simulink subsystem "BatteryManagementSystem"  (R2023b)
settings: Solver=VariableStepAuto  StartTime=0.0  StopTime=10.0  RelTol=1e-3
undefined symbols (not defined in the file or in its folder): battery, vehicleThermal
libraries: BatteryThermalManagement x1
settings Model: DefaultTestHarness=BatteryManagementSystem_Harness  Creator=jjha  LastModifiedBy=jjha
settings OptimizationCC: ReuseModelBlockBuffer=off

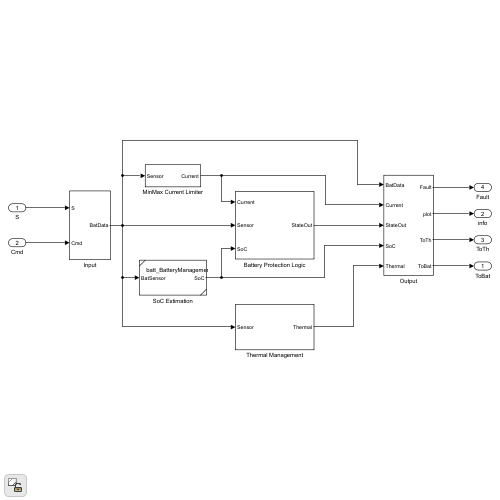
[thumbnail: Simulink's stored preview of the top-level diagram]
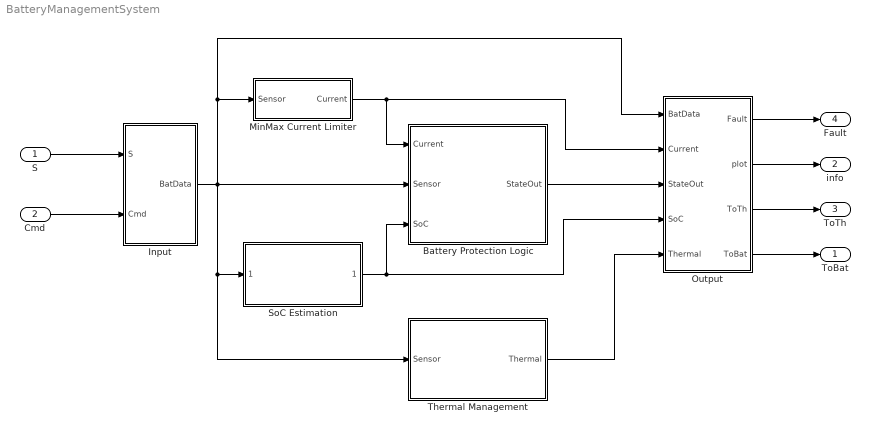
== system BatteryManagementSystem ==
  S : Inport
  Cmd : Inport  Port=2
  Battery Protection Logic : Subsystem
  Input : Subsystem
  MinMax Current Limiter : Subsystem
  Output : Subsystem
  SoC Estimation : Subsystem  ReferencedSubsystem=batt_BatteryManagementSystem_SoC
  Thermal Management : Subsystem
  ToBat : Outport
  info : Outport  Port=2
  ToTh : Outport  Port=3
  Fault : Outport  Port=4
  wires:
  Input/1(BatData) -> Battery Protection Logic/2(Sensor), SoC Estimation/1, Thermal Management/1(Sensor), Output/1(BatData), MinMax Current Limiter/1(Sensor)
  SoC Estimation/1 -> Battery Protection Logic/3(SoC), Output/4(SoC)
  Thermal Management/1(Thermal) -> Output/5(Thermal)
  MinMax Current Limiter/1(Current) -> Output/2(Current), Battery Protection Logic/1(Current)
  Battery Protection Logic/1(StateOut) -> Output/3(StateOut)
  S/1 -> Input/1(S)
  Output/1(Fault) -> Fault/1
  Output/2(plot) -> info/1
  Output/3(ToTh) -> ToTh/1
  Output/4(ToBat) -> ToBat/1
  Cmd/1 -> Input/2(Cmd)

== system BatteryManagementSystem/Battery Protection Logic ==
  Current : Inport
  Sensor : Inport  Port=2
  SoC : Inport  Port=3
  State Flow Logic : Subsystem  mask{MinVoltLmt=battery.MinVoltLmt, MaxVoltLmt=battery.MaxVoltLmt, VoltOffset=battery.VoltOffset, CurrOffset=battery.CurrOffset, MinThLmt=battery.MinThLmt, MaxThLmt=battery.MaxThLmt}
      mask prompts: MinVoltLmt "Minimum Voltage Limit"; MaxVoltLmt "Maximum Voltage Limit"; VoltOffset "Voltage fault offset"; CurrOffset "Current fault offset"; MinThLmt "Min cell temp"; MaxThLmt "Max cell temp"
      mask DialogControl ParameterGroupVar Prompt: Battery Fault Parameters
  Stateflow Input : Subsystem
  StateOut : Outport
  wires:
  State Flow Logic/1(StateOut) -> StateOut/1
  Stateflow Input/1(StateInput) -> State Flow Logic/1(StateInput)
  SoC/1 -> Stateflow Input/1(SoC)
  Current/1 -> Stateflow Input/2(Current)
  Sensor/1 -> Stateflow Input/3(Sensor)

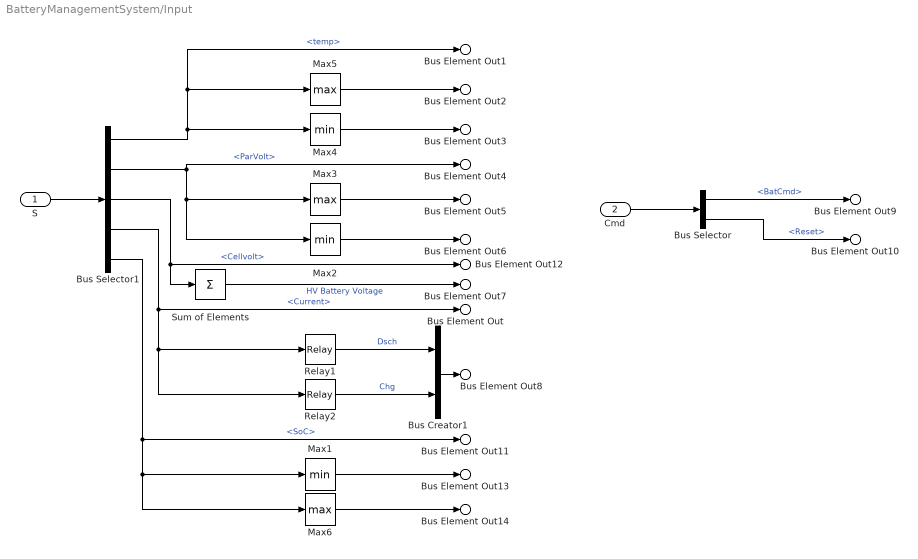
== system BatteryManagementSystem/Input ==
  S : Inport
  Cmd : Inport  Port=2
  Bus Creator1 : BusCreator  Inputs=2
  Bus Selector : BusSelector  OutputSignals=BatCmd,Reset
  Bus Selector1 : BusSelector  OutputSignals=temp,ParVolt,Cellvolt,Current,SoC
  Max1 : MinMax  ZeroCross=off
  Max2 : MinMax  ZeroCross=off
  Max3 : MinMax  Function=max  ZeroCross=off
  Max4 : MinMax  ZeroCross=off
  Max5 : MinMax  Function=max  ZeroCross=off
  Max6 : MinMax  Function=max  ZeroCross=off
  Relay1 : Relay  OnSwitchValue=0  OffSwitchValue=-5  OnOutputValue=0  OffOutputValue=1  ZeroCross=off
  Relay2 : Relay  OnSwitchValue=5  OffSwitchValue=0  ZeroCross=off
  Sum of Elements : Sum  Inputs=+
  Bus Element Out : Outport  PortName=BatData  Element=Cur
  Bus Element Out1 : Outport  PortName=BatData  Element=CellTemp
  Bus Element Out2 : Outport  PortName=BatData  Element=CellTempMax
  Bus Element Out3 : Outport  PortName=BatData  Element=CellTempMin
  Bus Element Out4 : Outport  PortName=BatData  Element=CellVolt
  Bus Element Out5 : Outport  PortName=BatData  Element=CellVoltMax
  Bus Element Out6 : Outport  PortName=BatData  Element=CellVoltMin
  Bus Element Out7 : Outport  PortName=BatData  Element=BatVolt
  Bus Element Out8 : Outport  PortName=BatData  Element=CurDir
  Bus Element Out11 : Outport  PortName=BatData  Element=SoC
  Bus Element Out12 : Outport  PortName=BatData  Element=BatParVolt
  Bus Element Out13 : Outport  PortName=BatData  Element=minSoC
  Bus Element Out14 : Outport  PortName=BatData  Element=maxSoC
  Bus Element Out9 : Outport  PortName=BatData  Element=BatCmd
  Bus Element Out10 : Outport  PortName=BatData  Element=Reset
  wires:
  Bus Selector/2 -> Bus Element Out10/1  "<Reset>"
  Cmd/1 -> Bus Selector/1
  Bus Selector/1 -> Bus Element Out9/1  "<BatCmd>"
  Bus Selector1/5 -> Bus Element Out11/1, Max1/1, Max6/1  "<SoC>"
  Bus Selector1/3 -> Sum of Elements/1, Bus Element Out12/1  "<Cellvolt>"
  Relay1/1 -> Bus Creator1/1  "Dsch"
  Bus Selector1/1 -> Bus Element Out1/1, Max5/1, Max4/1  "<temp>"
  Bus Selector1/4 -> Bus Element Out/1, Relay1/1, Relay2/1  "<Current>"
  Sum of Elements/1 -> Bus Element Out7/1  "HV Battery Voltage"
  S/1 -> Bus Selector1/1
  Bus Selector1/2 -> Bus Element Out4/1, Max3/1, Max2/1  "<ParVolt>"
  Max5/1 -> Bus Element Out2/1
  Max4/1 -> Bus Element Out3/1
  Max3/1 -> Bus Element Out5/1
  Max2/1 -> Bus Element Out6/1
  Bus Creator1/1 -> Bus Element Out8/1
  Relay2/1 -> Bus Creator1/2  "Chg"
  Max1/1 -> Bus Element Out13/1
  Max6/1 -> Bus Element Out14/1

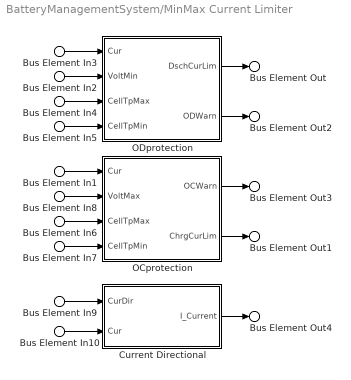
== system BatteryManagementSystem/MinMax Current Limiter ==
  Bus Element In3 : Inport  PortName=Sensor  Element=Cur
  Bus Element In1 : Inport  PortName=Sensor  Element=Cur
  Bus Element In10 : Inport  PortName=Sensor  Element=Cur
  Bus Element In2 : Inport  PortName=Sensor  Element=CellVoltMin
  Bus Element In8 : Inport  PortName=Sensor  Element=CellVoltMax
  Bus Element In9 : Inport  PortName=Sensor  Element=CurDir
  Bus Element In5 : Inport  PortName=Sensor  Element=CellTempMin
  Bus Element In7 : Inport  PortName=Sensor  Element=CellTempMin
  Bus Element In4 : Inport  PortName=Sensor  Element=CellTempMax
  Bus Element In6 : Inport  PortName=Sensor  Element=CellTempMax
  Current Directional : Subsystem
  OCprotection : Subsystem
  ODprotection : Subsystem
  Bus Element Out : Outport  PortName=Current  Element=CurDchLmt
  Bus Element Out1 : Outport  PortName=Current  Element=CurChgLmt
  Bus Element Out2 : Outport  PortName=Current  Element=CurDchWarn
  Bus Element Out3 : Outport  PortName=Current  Element=CurChgWarn
  Bus Element Out4 : Outport  PortName=Current  Element=CurChgDchg
  wires:
  ODprotection/2(ODWarn) -> Bus Element Out2/1
  Bus Element In8/1 -> OCprotection/2(VoltMax)
  Bus Element In2/1 -> ODprotection/2(VoltMin)
  OCprotection/1(OCWarn) -> Bus Element Out3/1
  Bus Element In6/1 -> OCprotection/3(CellTpMax)
  Bus Element In7/1 -> OCprotection/4(CellTpMin)
  Bus Element In9/1 -> Current Directional/1(CurDir)
  Bus Element In4/1 -> ODprotection/3(CellTpMax)
  Bus Element In5/1 -> ODprotection/4(CellTpMin)
  ODprotection/1(DschCurLim) -> Bus Element Out/1
  OCprotection/2(ChrgCurLim) -> Bus Element Out1/1
  Bus Element In3/1 -> ODprotection/1(Cur)
  Bus Element In1/1 -> OCprotection/1(Cur)
  Current Directional/1(I_Current) -> Bus Element Out4/1
  Bus Element In10/1 -> Current Directional/2(Cur)

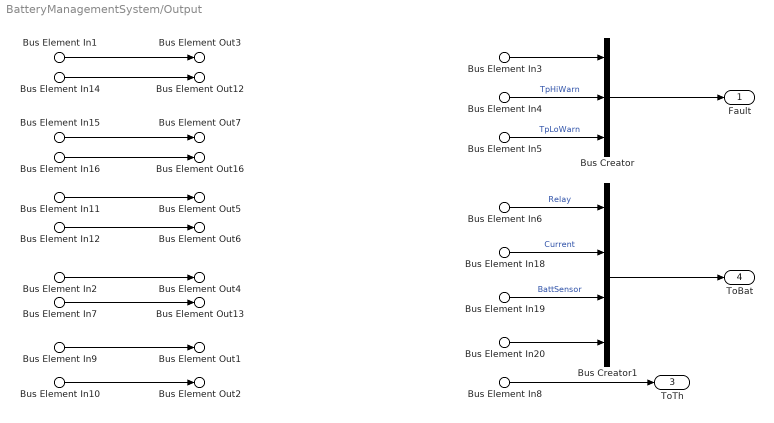
== system BatteryManagementSystem/Output ==
  Bus Element In19 : Inport  PortName=BatData
  Bus Element In9 : Inport  PortName=BatData  Element=Cur
  Bus Element In10 : Inport  PortName=BatData  Element=BatVolt
  Bus Element In11 : Inport  PortName=BatData  Element=CellTempMax
  Bus Element In12 : Inport  PortName=BatData  Element=CellTempMin
  Bus Element In18 : Inport  Port=2  PortName=Current
  Bus Element In2 : Inport  Port=2  PortName=Current  Element=CurChgLmt
  Bus Element In7 : Inport  Port=2  PortName=Current  Element=CurDchLmt
  Bus Element In3 : Inport  Port=3  PortName=StateOut  Element=Fault
  Bus Element In6 : Inport  Port=3  PortName=StateOut  Element=RelayRq
  Bus Element In20 : Inport  Port=3  PortName=StateOut  Element=BatSt
  Bus Element In1 : Inport  Port=4  PortName=SoC  Element=CellSoCmax
  Bus Element In14 : Inport  Port=4  PortName=SoC  Element=CellSoCmin
  Bus Element In8 : Inport  Port=5  PortName=Thermal
  Bus Element In{4..5,15..16} (4 alike) : Inport  Port=5  PortName=Thermal  Element=TpHiWarning
  Bus Creator : BusCreator  Inputs=3
  Bus Creator1 : BusCreator  Inputs=4
  Fault : Outport
  Bus Element Out3 : Outport  Port=2  PortName=plot  Element=SoCMax
  Bus Element Out4 : Outport  Port=2  PortName=plot  Element=CurChgLmt
  Bus Element Out7 : Outport  Port=2  PortName=plot  Element=HiThWarn
  Bus Element Out12 : Outport  Port=2  PortName=plot  Element=SoCMin
  Bus Element Out13 : Outport  Port=2  PortName=plot  Element=CurDchgLmt
  Bus Element Out16 : Outport  Port=2  PortName=plot  Element=LoThWarn
  Bus Element Out1 : Outport  Port=2  PortName=plot  Element=Cur
  Bus Element Out2 : Outport  Port=2  PortName=plot  Element=BatVolt
  Bus Element Out5 : Outport  Port=2  PortName=plot  Element=TpMax
  Bus Element Out6 : Outport  Port=2  PortName=plot  Element=TpMin
  ToTh : Outport  Port=3
  ToBat : Outport  Port=4
  wires:
  Bus Element In8/1 -> ToTh/1
  Bus Creator/1 -> Fault/1
  Bus Creator1/1 -> ToBat/1
  Bus Element In18/1 -> Bus Creator1/2  "Current"
  Bus Element In12/1 -> Bus Element Out6/1
  Bus Element In11/1 -> Bus Element Out5/1
  Bus Element In10/1 -> Bus Element Out2/1
  Bus Element In9/1 -> Bus Element Out1/1
  Bus Element In6/1 -> Bus Creator1/1  "Relay"
  Bus Element In5/1 -> Bus Creator/3  "TpLoWarn"
  Bus Element In4/1 -> Bus Creator/2  "TpHiWarn"
  Bus Element In3/1 -> Bus Creator/1
  Bus Element In14/1 -> Bus Element Out12/1
  Bus Element In2/1 -> Bus Element Out4/1
  Bus Element In1/1 -> Bus Element Out3/1
  Bus Element In7/1 -> Bus Element Out13/1
  Bus Element In15/1 -> Bus Element Out7/1
  Bus Element In16/1 -> Bus Element Out16/1
  Bus Element In19/1 -> Bus Creator1/3  "BattSensor"
  Bus Element In20/1 -> Bus Creator1/4

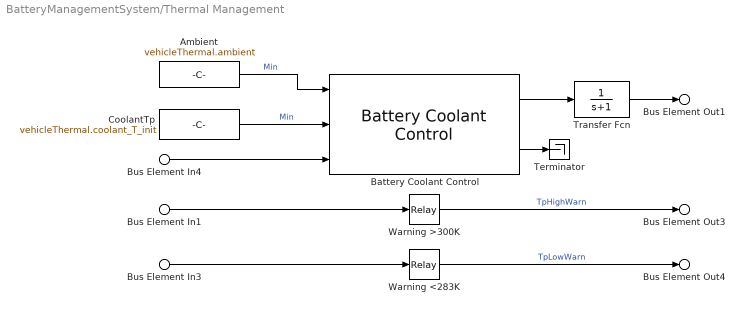
== system BatteryManagementSystem/Thermal Management ==
  Bus Element In3 : Inport  PortName=Sensor  Element=CellTempMin
  Bus Element In1 : Inport  PortName=Sensor  Element=CellTempMax
  Bus Element In4 : Inport  PortName=Sensor  Element=CellTemp
  Ambient : Constant  Value=vehicleThermal.ambient
  Battery Coolant Control : BatteryThermalManagement/Battery Coolant Control  ControlStrategy=ON-OFF control  TempOn=battery.CoolantSwitchOnTp  TempOff=battery.CoolantSwitchOffTp  c=0.1  FlowRateStep=0.2
      settings: LibrarySourceBlock=batt_sl_lib/Thermal Management/Battery Coolant Control
  CoolantTp : Constant  Value=vehicleThermal.coolant_T_init
  Terminator : Terminator
  Transfer Fcn : TransferFcn  Denominator=[1 1]
  Warning <283K : Relay  OnSwitchValue=290  OffSwitchValue=283  OnOutputValue=0  OffOutputValue=1  ZeroCross=off
  Warning >300K : Relay  OnSwitchValue=320  OffSwitchValue=310  ZeroCross=off
  Bus Element Out1 : Outport  PortName=Thermal  Element=CoolFlow
  Bus Element Out3 : Outport  PortName=Thermal  Element=TpHiWarning
  Bus Element Out4 : Outport  PortName=Thermal  Element=TpLoWarning
  wires:
  Battery Coolant Control/2 -> Terminator/1
  Bus Element In4/1 -> Battery Coolant Control/3
  Transfer Fcn/1 -> Bus Element Out1/1
  CoolantTp/1 -> Battery Coolant Control/2  "Min"
  Ambient/1 -> Battery Coolant Control/1  "Min"
  Bus Element In3/1 -> Warning <283K/1
  Bus Element In1/1 -> Warning >300K/1
  Warning <283K/1 -> Bus Element Out4/1  "TpLowWarn"
  Warning >300K/1 -> Bus Element Out3/1  "TpHighWarn"
  Battery Coolant Control/1 -> Transfer Fcn/1

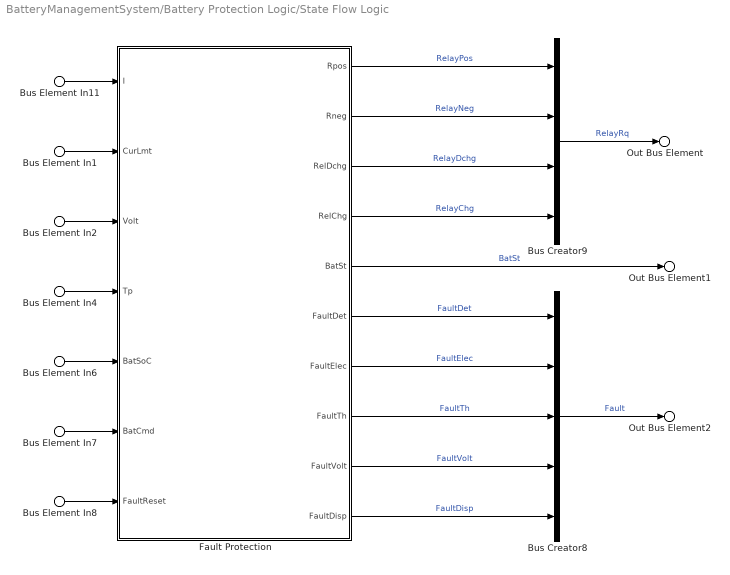
== system BatteryManagementSystem/Battery Protection Logic/State Flow Logic ==
  Bus Element In11 : Inport  PortName=StateInput  Element=Current
  Bus Element In1 : Inport  PortName=StateInput  Element=CurLmt
  Bus Element In2 : Inport  PortName=StateInput  Element=Volt
  Bus Element In4 : Inport  PortName=StateInput  Element=Tp
  Bus Element In6 : Inport  PortName=StateInput  Element=BatSoC
  Bus Element In7 : Inport  PortName=StateInput  Element=BatCmd
  Bus Element In8 : Inport  PortName=StateInput  Element=FaultReset
  Bus Creator8 : BusCreator  Inputs=5
  Bus Creator9 : BusCreator  Inputs=4
  Fault Protection : Stateflow chart  TreatAsAtomicUnit=on
      settings: PortSchema="{\"entries\":[{\"content\":{\"sides\":[{\"content\":{\"connectorIds\":[\"In1\",\"In2\",\"In3\",\"In4\",\"In5\",\"In6\",\"In7\"]},\"type\":\"ConnectorPlacement.EquallySpacedRectSide\",\"uuid\":\"7222f55a-2aef-4ca8-adbd-e86ed030f82f\"},{\"content\":{\"connectorIds\":[\"Out5\",\"Out6\",\"Out10\",\"Out9\",\"Out4\",\"Out1\",\"Out2\",\"Out3\",\"Out7\",\"Out8\"],\"side\":\"RIGHT\"},\"type\":\"ConnectorPlacement.EquallySpacedRectSide\",\"uuid\":\"bfa2f4e3-3563-4466-8725-57bf2336ec66\"},{\"content\":{\"connectorIds\":[],\"side\":\"TOP\"},\"type\":\"ConnectorPlacement.EquallySpacedRectSide\",\"uuid\":\"7b1e9a44-7135-4c45-bb2b-0152be29b46d\"}]},\"type\":\"ConnectorPlacement.EquallySpacedConnector\",\"uuid\":\"80032a24-3823-40c6-b797-ffbc29f7d345\"}],\"packageUris\":[\"http://schema.mathworks.com/mf0/Connector/R2020b\"],\"version\":\"1.0\"}"
  Out Bus Element : Outport  PortName=StateOut  Element=RelayRq
  Out Bus Element1 : Outport  PortName=StateOut  Element=BatSt
  Out Bus Element2 : Outport  PortName=StateOut  Element=Fault
  wires:
  Fault Protection/4(BatSt) -> Out Bus Element1/1  "BatSt"
  Fault Protection/9(RelChg) -> Bus Creator9/4  "RelayChg"
  Fault Protection/10(RelDchg) -> Bus Creator9/3  "RelayDchg"
  Fault Protection/6(Rneg) -> Bus Creator9/2  "RelayNeg"
  Fault Protection/5(Rpos) -> Bus Creator9/1  "RelayPos"
  Bus Element In7/1 -> Fault Protection/6(BatCmd)
  Bus Element In8/1 -> Fault Protection/7(FaultReset)
  Bus Element In2/1 -> Fault Protection/3(Volt)
  Bus Element In1/1 -> Fault Protection/2(CurLmt)
  Bus Element In11/1 -> Fault Protection/1(I)
  Bus Element In4/1 -> Fault Protection/4(Tp)
  Bus Element In6/1 -> Fault Protection/5(BatSoC)
  Bus Creator9/1 -> Out Bus Element/1  "RelayRq"
  Bus Creator8/1 -> Out Bus Element2/1  "Fault"
  Fault Protection/2(FaultElec) -> Bus Creator8/2  "FaultElec"
  Fault Protection/3(FaultTh) -> Bus Creator8/3  "FaultTh"
  Fault Protection/7(FaultVolt) -> Bus Creator8/4  "FaultVolt"
  Fault Protection/8(FaultDisp) -> Bus Creator8/5  "FaultDisp"
  Fault Protection/1(FaultDet) -> Bus Creator8/1  "FaultDet"

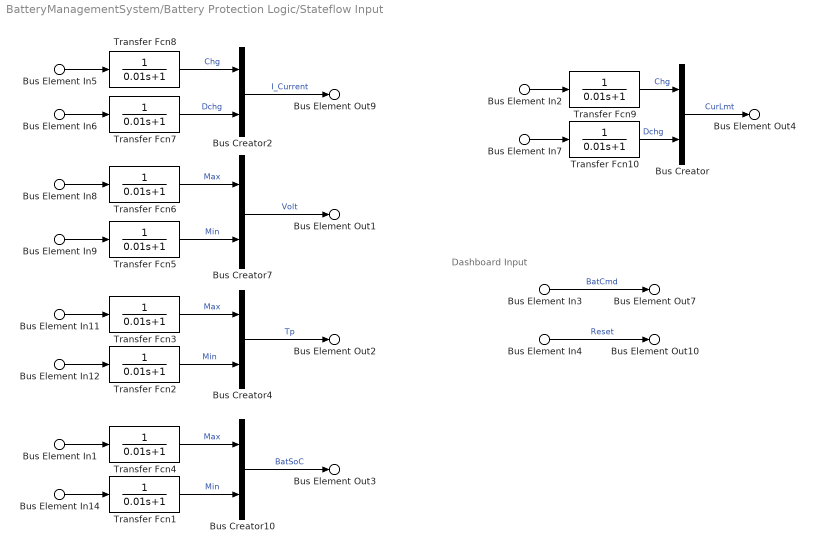
== system BatteryManagementSystem/Battery Protection Logic/Stateflow Input ==
  note: Dashboard Input
  Bus Element In1 : Inport  PortName=SoC  Element=CellSoCmax
  Bus Element In14 : Inport  PortName=SoC  Element=CellSoCmin
  Bus Element In2 : Inport  Port=2  PortName=Current  Element=CurChgLmt
  Bus Element In7 : Inport  Port=2  PortName=Current  Element=CurDchLmt
  Bus Element In5 : Inport  Port=2  PortName=Current  Element=CurChgDchg.Chg
  Bus Element In6 : Inport  Port=2  PortName=Current  Element=CurChgDchg.Dchg
  Bus Element In8 : Inport  Port=3  PortName=Sensor  Element=CellVoltMax
  Bus Element In9 : Inport  Port=3  PortName=Sensor  Element=CellVoltMin
  Bus Element In11 : Inport  Port=3  PortName=Sensor  Element=CellTempMax
  Bus Element In12 : Inport  Port=3  PortName=Sensor  Element=CellTempMin
  Bus Element In3 : Inport  Port=3  PortName=Sensor  Element=BatCmd
  Bus Element In4 : Inport  Port=3  PortName=Sensor  Element=Reset
  Bus Creator : BusCreator  Inputs=2  OutDataTypeStr=Bus: I_Current
  Bus Creator10 : BusCreator  Inputs=2  OutDataTypeStr=Bus: MaxMinLimit
  Bus Creator2 : BusCreator  Inputs=2  OutDataTypeStr=Bus: I_Current
  Bus Creator4 : BusCreator  Inputs=2  OutDataTypeStr=Bus: MaxMinLimit
  Bus Creator7 : BusCreator  Inputs=2  OutDataTypeStr=Bus: CellVoltage  NonVirtualBus=on
  Transfer Fcn{1..10} (10 alike) : TransferFcn  Denominator=[0.01 1]
  Bus Element Out9 : Outport  PortName=StateInput  Element=Current
  Bus Element Out1 : Outport  PortName=StateInput  Element=Volt
  Bus Element Out2 : Outport  PortName=StateInput  Element=Tp
  Bus Element Out3 : Outport  PortName=StateInput  Element=BatSoC
  Bus Element Out4 : Outport  PortName=StateInput  Element=CurLmt
  Bus Element Out7 : Outport  PortName=StateInput  Element=BatCmd
  Bus Element Out10 : Outport  PortName=StateInput  Element=FaultReset
  wires:
  Transfer Fcn10/1 -> Bus Creator/2  "Dchg"
  Transfer Fcn9/1 -> Bus Creator/1  "Chg"
  Transfer Fcn7/1 -> Bus Creator2/2  "Dchg"
  Transfer Fcn8/1 -> Bus Creator2/1  "Chg"
  Transfer Fcn6/1 -> Bus Creator7/1  "Max"
  Transfer Fcn5/1 -> Bus Creator7/2  "Min"
  Transfer Fcn3/1 -> Bus Creator4/1  "Max"
  Transfer Fcn2/1 -> Bus Creator4/2  "Min"
  Transfer Fcn1/1 -> Bus Creator10/2  "Min"
  Transfer Fcn4/1 -> Bus Creator10/1  "Max"
  Bus Element In7/1 -> Transfer Fcn10/1
  Bus Element In2/1 -> Transfer Fcn9/1
  Bus Creator7/1 -> Bus Element Out1/1  "Volt"
  Bus Creator2/1 -> Bus Element Out9/1  "I_Current"
  Bus Creator4/1 -> Bus Element Out2/1  "Tp"
  Bus Element In3/1 -> Bus Element Out7/1  "BatCmd"
  Bus Element In4/1 -> Bus Element Out10/1  "Reset"
  Bus Element In14/1 -> Transfer Fcn1/1
  Bus Element In1/1 -> Transfer Fcn4/1
  Bus Element In6/1 -> Transfer Fcn7/1
  Bus Element In5/1 -> Transfer Fcn8/1
  Bus Creator10/1 -> Bus Element Out3/1  "BatSoC"
  Bus Element In11/1 -> Transfer Fcn3/1
  Bus Creator/1 -> Bus Element Out4/1  "CurLmt"
  Bus Element In9/1 -> Transfer Fcn5/1
  Bus Element In8/1 -> Transfer Fcn6/1
  Bus Element In12/1 -> Transfer Fcn2/1

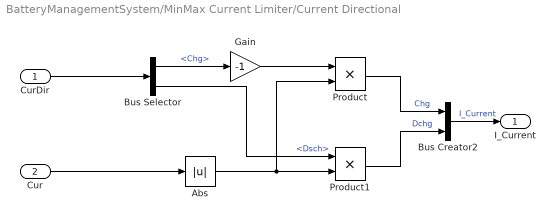
== system BatteryManagementSystem/MinMax Current Limiter/Current Directional ==
  CurDir : Inport
  Cur : Inport  Port=2
  Abs : Abs  ZeroCross=off  SaturateOnIntegerOverflow=off
  Bus Creator2 : BusCreator  Inputs=2  OutDataTypeStr=Bus: I_Current
  Bus Selector : BusSelector  OutputSignals=Chg,Dsch
  Gain : Gain  Gain=-1
  Product : Product
  Product1 : Product
  I_Current : Outport
  wires:
  Gain/1 -> Product/1
  Cur/1 -> Abs/1
  Abs/1 -> Product/2, Product1/2
  CurDir/1 -> Bus Selector/1
  Bus Selector/1 -> Gain/1  "<Chg>"
  Bus Selector/2 -> Product1/1  "<Dsch>"
  Product/1 -> Bus Creator2/1  "Chg"
  Bus Creator2/1 -> I_Current/1  "I_Current"
  Product1/1 -> Bus Creator2/2  "Dchg"

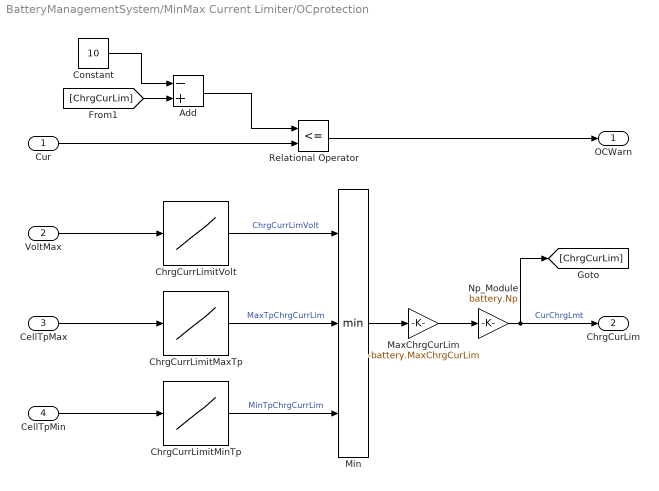
== system BatteryManagementSystem/MinMax Current Limiter/OCprotection ==
  Cur : Inport
  VoltMax : Inport  Port=2
  CellTpMax : Inport  Port=3
  CellTpMin : Inport  Port=4
  Add : Sum  Inputs=-+
  ChrgCurrLimitMaxTp : Lookup_n-D  NumberOfTableDimensions=1  BreakpointsForDimension1="single([313  318  323  328 333])"  BreakpointsForDimension3=[5, 7]  Table=single([1.0 0.8 0.5 0.3 0])  ExtrapMethod=Clip  UseLastTableValue=on  InternalRulePriority=Speed  RndMeth=Simplest
  ChrgCurrLimitMinTp : Lookup_n-D  NumberOfTableDimensions=1  BreakpointsForDimension1=single([258 263 268 273 278 283 288])  BreakpointsForDimension3=[5, 7]  Table="single([0.1 0.2  0.3 0.3 0.5 1.0 1.0])"  ExtrapMethod=Clip  UseLastTableValue=on  InternalRulePriority=Speed  RndMeth=Simplest
  ChrgCurrLimitVolt : Lookup_n-D  NumberOfTableDimensions=1  BreakpointsForDimension1=single([3.9 4.0 4.15 4.2])  BreakpointsForDimension3=[5, 7]  Table="single([1.0 0.8 0.3  0.3])"  ExtrapMethod=Clip  UseLastTableValue=on  InternalRulePriority=Speed  RndMeth=Simplest
  Constant : Constant  Value=10
  MaxChrgCurLim : Gain  Gain=-battery.MaxChrgCurLim
  Min : MinMax  Inputs=3
  Np_Module : Gain  Gain=battery.Np
  Relational Operator : RelationalOperator  Operator=<=  OutDataTypeStr=boolean  RndMeth=Simplest  InputSameDT=off
  OCWarn : Outport
  ChrgCurLim : Outport  Port=2
  wires:
  Add/1 -> Relational Operator/1
  Constant/1 -> Add/1
  VoltMax/1 -> ChrgCurrLimitVolt/1
  ChrgCurrLimitVolt/1 -> Min/1  "ChrgCurrLimVolt"
  MaxChrgCurLim/1 -> Np_Module/1
  Np_Module/1 -> ChrgCurLim/1, [ChrgCurLim]  "CurChrgLmt"
  CellTpMax/1 -> ChrgCurrLimitMaxTp/1
  CellTpMin/1 -> ChrgCurrLimitMinTp/1
  ChrgCurrLimitMaxTp/1 -> Min/2  "MaxTpChrgCurrLim"
  ChrgCurrLimitMinTp/1 -> Min/3  "MinTpChrgCurrLim"
  Min/1 -> MaxChrgCurLim/1
  Cur/1 -> Relational Operator/2
  [ChrgCurLim] -> Add/2
  Relational Operator/1 -> OCWarn/1

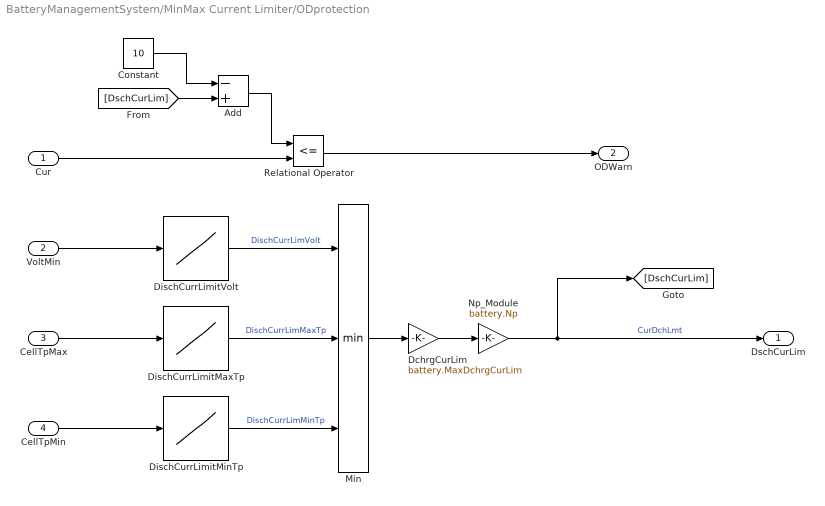
== system BatteryManagementSystem/MinMax Current Limiter/ODprotection ==
  Cur : Inport
  VoltMin : Inport  Port=2
  CellTpMax : Inport  Port=3
  CellTpMin : Inport  Port=4
  Add : Sum  Inputs=-+
  Constant : Constant  Value=10
  DchrgCurLim : Gain  Gain=battery.MaxDchrgCurLim
  DischCurrLimitMaxTp : Lookup_n-D  NumberOfTableDimensions=1  BreakpointsForDimension1=single([313, 318, 323, 333])  BreakpointsForDimension3=[5, 7]  Table=single([1, 0.5, 0.3, 0])  ExtrapMethod=Clip  UseLastTableValue=on  InternalRulePriority=Speed  RndMeth=Simplest
  DischCurrLimitMinTp : Lookup_n-D  NumberOfTableDimensions=1  BreakpointsForDimension1="single([263, 268,    273,   278, 283, 288, 293])"  BreakpointsForDimension3=[5, 7]  Table="single([0,  0.2, 0.3, 0.5, 0.75, 1, 1])"  ExtrapMethod=Clip  UseLastTableValue=on  InternalRulePriority=Speed  RndMeth=Simplest
  DischCurrLimitVolt : Lookup_n-D  NumberOfTableDimensions=1  BreakpointsForDimension1=single([2.5;3;3.5;4.2])  BreakpointsForDimension3=[5, 7]  Table=single([0 0.25 0.5 0.75])  ExtrapMethod=Clip  UseLastTableValue=on  InternalRulePriority=Speed  RndMeth=Simplest
  Min : MinMax  Inputs=3
  Np_Module : Gain  Gain=battery.Np
  Relational Operator : RelationalOperator  Operator=<=  OutDataTypeStr=boolean  RndMeth=Simplest  InputSameDT=off
  DschCurLim : Outport
  ODWarn : Outport  Port=2
  wires:
  Constant/1 -> Add/1
  Add/1 -> Relational Operator/1
  Relational Operator/1 -> ODWarn/1
  [DschCurLim] -> Add/2
  Cur/1 -> Relational Operator/2
  Min/1 -> DchrgCurLim/1
  DischCurrLimitMinTp/1 -> Min/3  "DischCurrLimMinTp"
  DischCurrLimitMaxTp/1 -> Min/2  "DischCurrLimMaxTp"
  CellTpMax/1 -> DischCurrLimitMaxTp/1
  Np_Module/1 -> [DschCurLim], DschCurLim/1  "CurDchLmt"
  DchrgCurLim/1 -> Np_Module/1
  DischCurrLimitVolt/1 -> Min/1  "DischCurrLimVolt"
  VoltMin/1 -> DischCurrLimitVolt/1
  CellTpMin/1 -> DischCurrLimitMinTp/1

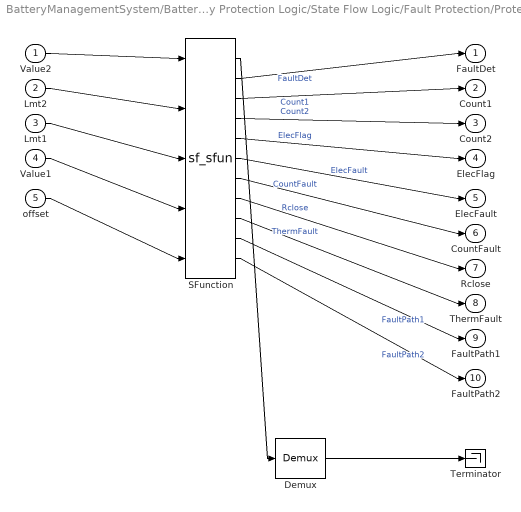
== system BatteryManagementSystem/Battery Protection Logic/State Flow Logic/Fault Protection/Protection.CurrFault ==
  Value2 : Inport
  Lmt2 : Inport  Port=2
  Lmt1 : Inport  Port=3
  Value1 : Inport  Port=4
  offset : Inport  Port=5
  " Demux " : Demux  Outputs=1
  " SFunction " : S-Function  Tag=Stateflow S-Function 3  FunctionName=sf_sfun  PortCounts=[5 11]  SFunctionDeploymentMode=off  EnableBusSupport=off
  " Terminator " : Terminator
  FaultDet : Outport
  Count1 : Outport  Port=2
  Count2 : Outport  Port=3
  ElecFlag : Outport  Port=4
  ElecFault : Outport  Port=5
  CountFault : Outport  Port=6
  Rclose : Outport  Port=7
  ThermFault : Outport  Port=8
  FaultPath1 : Outport  Port=9
  FaultPath2 : Outport  Port=10
  wires:
  Value2/1 -> " SFunction "/1
  Lmt2/1 -> " SFunction "/2
  Lmt1/1 -> " SFunction "/3
  Value1/1 -> " SFunction "/4
  offset/1 -> " SFunction "/5
  " SFunction "/2 -> FaultDet/1  "FaultDet"
  " SFunction "/3 -> Count1/1  "Count1"
  " SFunction "/4 -> Count2/1  "Count2"
  " SFunction "/5 -> ElecFlag/1  "ElecFlag"
  " SFunction "/6 -> ElecFault/1  "ElecFault"
  " SFunction "/7 -> CountFault/1  "CountFault"
  " SFunction "/8 -> Rclose/1  "Rclose"
  " SFunction "/9 -> ThermFault/1  "ThermFault"
  " SFunction "/10 -> FaultPath1/1  "FaultPath1"
  " SFunction "/11 -> FaultPath2/1  "FaultPath2"
  " Demux "/1 -> " Terminator "/1
  " SFunction "/1 -> " Demux "/1

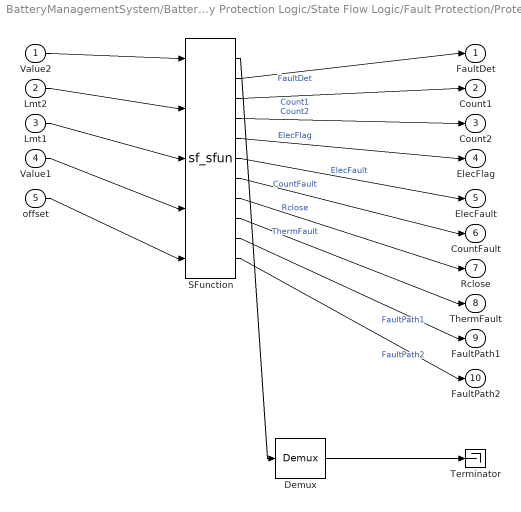
== system BatteryManagementSystem/Battery Protection Logic/State Flow Logic/Fault Protection/Protection.VoltageFault ==
  Value2 : Inport
  Lmt2 : Inport  Port=2
  Lmt1 : Inport  Port=3
  Value1 : Inport  Port=4
  offset : Inport  Port=5
  " Demux " : Demux  Outputs=1
  " SFunction " : S-Function  Tag=Stateflow S-Function 5  FunctionName=sf_sfun  PortCounts=[5 11]  SFunctionDeploymentMode=off  EnableBusSupport=off
  " Terminator " : Terminator
  FaultDet : Outport
  Count1 : Outport  Port=2
  Count2 : Outport  Port=3
  ElecFlag : Outport  Port=4
  ElecFault : Outport  Port=5
  CountFault : Outport  Port=6
  Rclose : Outport  Port=7
  ThermFault : Outport  Port=8
  FaultPath1 : Outport  Port=9
  FaultPath2 : Outport  Port=10
  wires:
  Value2/1 -> " SFunction "/1
  Lmt2/1 -> " SFunction "/2
  Lmt1/1 -> " SFunction "/3
  Value1/1 -> " SFunction "/4
  offset/1 -> " SFunction "/5
  " SFunction "/2 -> FaultDet/1  "FaultDet"
  " SFunction "/3 -> Count1/1  "Count1"
  " SFunction "/4 -> Count2/1  "Count2"
  " SFunction "/5 -> ElecFlag/1  "ElecFlag"
  " SFunction "/6 -> ElecFault/1  "ElecFault"
  " SFunction "/7 -> CountFault/1  "CountFault"
  " SFunction "/8 -> Rclose/1  "Rclose"
  " SFunction "/9 -> ThermFault/1  "ThermFault"
  " SFunction "/10 -> FaultPath1/1  "FaultPath1"
  " SFunction "/11 -> FaultPath2/1  "FaultPath2"
  " Demux "/1 -> " Terminator "/1
  " SFunction "/1 -> " Demux "/1

== system BatteryManagementSystem/Battery Protection Logic/State Flow Logic/Fault Protection/Relay_Charge ==
  " Demux " : Demux  Outputs=1
  " Ground " : Ground
  " SFunction " : S-Function  Tag=Stateflow S-Function 6  FunctionName=sf_sfun  PortCounts=[1 5]  SFunctionDeploymentMode=off  EnableBusSupport=off
  " Terminator " : Terminator
  RelClosing : Outport
  RelClose : Outport  Port=2
  Relay : Outport  Port=3
  RelOpening : Outport  Port=4
  wires:
  " SFunction "/2 -> RelClosing/1  "RelClosing"
  " SFunction "/3 -> RelClose/1  "RelClose"
  " SFunction "/4 -> Relay/1  "Relay"
  " SFunction "/5 -> RelOpening/1  "RelOpening"
  " Ground "/1 -> " SFunction "/1
  " Demux "/1 -> " Terminator "/1
  " SFunction "/1 -> " Demux "/1

== system BatteryManagementSystem/Battery Protection Logic/State Flow Logic/Fault Protection/Relay_Discharge ==
  " Demux " : Demux  Outputs=1
  " Ground " : Ground
  " SFunction " : S-Function  Tag=Stateflow S-Function 7  FunctionName=sf_sfun  PortCounts=[1 5]  SFunctionDeploymentMode=off  EnableBusSupport=off
  " Terminator " : Terminator
  RelClosing : Outport
  RelClose : Outport  Port=2
  Relay : Outport  Port=3
  RelOpening : Outport  Port=4
  wires:
  " SFunction "/2 -> RelClosing/1  "RelClosing"
  " SFunction "/3 -> RelClose/1  "RelClose"
  " SFunction "/4 -> Relay/1  "Relay"
  " SFunction "/5 -> RelOpening/1  "RelOpening"
  " Ground "/1 -> " SFunction "/1
  " Demux "/1 -> " Terminator "/1
  " SFunction "/1 -> " Demux "/1

== stateflow chart BatteryManagementSystem/Battery Protection Logic/State Flow Logic/Fault Protection ==
  state BatteryRequest [parallel]
    settings: executionOrder=1
    state BatteryConnect_Req
      BatReq=1;
    state BatteryDischarging
      BatSt=3;
    state Standby
      BatSt=0;
    state OpenDchg
      RelDchgOpening=1;
    state BatteryDchgReq
      BatReq=3;
      RelDchgClosing=1;
    state Battery_Connect
      Rclosing=1;
    state Idle_State
      BatSt=1;
    state OpenChg
      RelChgOpening=1;
    state Battery_disconnect
      BatReq=0;
      Ropening=1;
      BatSt=0.25;
    state BatteryChgReq
      BatReq=2;
      RelChgClosing=1;
    state BatteryCharging
      BatSt=2;
    (default) -> Standby : {BatReq=0;Rpos=0; Rneg=0;
        |  Rclosing=0;Ropening=0;
        | RelChgOpening=0;RelChgClosing=0;
        | RelDchgOpening=0;RelDchgClosing=0;}
    BatteryDischarging -> BatteryConnect_Req : [BatCmd~=3 || BatSoC.Min<0.01 || FaultDet==1]
    BatteryConnect_Req -> OpenDchg [order 2] : [BatSt==3]
    Standby -> BatteryConnect_Req : [BatCmd~=0 && BatSoC.Min>=0.05 ...
        | && FaultDet==0 && CountFault==0]
    OpenDchg -> Idle_State : [RelDchgClose==0]
    Battery_disconnect -> Standby : [Rclose==0]
    BatteryDchgReq -> BatteryDischarging : [RelDchgClose==1]
    Idle_State -> BatteryDchgReq [order 1] : [BatCmd==3 && FaultDet==0 ...
        | &&  BatSoC.Min>=0.05]
    BatteryConnect_Req -> Battery_Connect [order 1] : [ FaultDet==0 ...
        | && CountFault==0 ...
        | && BatSt==0]
    Battery_Connect -> Idle_State : [Rclose==1]
    BatteryCharging -> BatteryConnect_Req : [BatCmd~=2 || BatSoC.Max>0.99 ...
        | || FaultDet==1]
    BatteryConnect_Req -> (junction 399) [order 3] : [BatSt==2]
    (junction 399) -> OpenChg
    Idle_State -> (junction 392) [order 2] : [BatCmd==0 || BatSoC.Min<=0.01 ...
        |  || BatSoC.Min>=0.99 || FaultDet==1]
    OpenChg -> Idle_State : [RelChgClose==0]
    (junction 392) -> (junction 393)
    Idle_State -> BatteryChgReq [order 3] : [BatCmd==2 ...
        | && BatSoC.Max<=0.97 ...
        |  && FaultDet==0 ]
    (junction 394) -> Battery_disconnect
    BatteryChgReq -> (junction 113) : [RelChgClose==1]
    (junction 113) -> BatteryCharging
    (junction 393) -> (junction 394)
  state Protection [group]
    state ThermalFault [parallel]
      settings: executionOrder=1
      state NoFault
      state DebounceMin
      state FaultDetected
        FaultDet=1;
        FaultDisp.ThermFault=1;
      state DebounceMax
      (default) -> NoFault : {FaultDet=0;
          | FaultTh.Min=0;
          | FaultTh.Max=0;
          | ThermFault=0;}
      DebounceMin -> NoFault [order 1] : [Tp.Min>MinThLmt]
      NoFault -> DebounceMin [order 1] : [Tp.Min<MinThLmt ...
          | && Rclose==1]
      DebounceMin -> FaultDetected [order 2] : after(10,sec)
          | {FaultTh.Min=1;}
      NoFault -> DebounceMax [order 2] : [Tp.Max>MaxThLmt ...
          | && Rclose==1]
      DebounceMax -> FaultDetected [order 2] : after(10,sec)
          | {FaultTh.Max=1;}
      DebounceMax -> NoFault [order 1] : [Tp.Max<MaxThLmt]
    state CurrFault [parallel]
      settings: executionOrder=4
    state VoltageFault [parallel]
      settings: executionOrder=3
    state Reset [parallel]
      settings: executionOrder=2
      state Reset
        CountFault=0;
        VoltFault=0;
        ElecFault=0;
        FaultDet=0;
        FaultDisp.VoltFault=0;
        FaultDisp.CountMin=0;CountMin=0;
        FaultDisp.CountMax=0;CountMax=0;
        FaultDisp.CurrFault=0;
        FaultDisp.CountCh=0;CountCh=0;
        FaultDisp.CountDch=0;CountDch=0;
      state Wait
      (default) -> Wait
      Wait -> Protection.Reset.Reset : [FaultReset==1]
      Protection.Reset.Reset -> Wait : [FaultReset==0]
  state RelayOperationBattery [parallel]
    settings: executionOrder=2
    state RelayOpen
      state PosRelayOpen
        Rpos=0;
      state NegRelayOpen
        Rneg=0;
      state Opened
        Rclose=0;
        Ropening=0;
      (default) -> PosRelayOpen
      PosRelayOpen -> NegRelayOpen : after(100,msec)
      NegRelayOpen -> Opened : after(100,msec)
    state RelayClose
      state NegRelayClose
        Rneg=1;
        Rclose=0;
      state PosRelayClose
        Rpos=1;
      state Closed
        Rclose=1;
        Rclosing=0;
      (default) -> NegRelayClose
      NegRelayClose -> PosRelayClose : after(100,msec)
      PosRelayClose -> Closed : after(100,msec)
    (default) -> RelayOpen : {Rneg=0; Rpos=0;
        | Rclose=0;}
    Opened -> RelayClose : [Rclosing==1]
    Closed -> RelayOpen : [Ropening==1]
  state Relay_Discharge [parallel]
    settings: executionOrder=3
  state Relay_Charge [parallel]
    settings: executionOrder=4
  data: Count1 function_output; Value2 function_input; Count2 function_output; ElecFlag function_output; ElecFault function_output; CountFault function_output; Rclose function_output; ThermFault function_output; Lmt2 function_input; Lmt1 function_input; Value1 function_input; FaultPath1 function_output; FaultPath2 function_output; offset function_input; Count1 function_output; Value2 function_input; Count2 function_output; ElecFlag function_output; ElecFault function_output; CountFault function_output; Rclose function_output; ThermFault function_output; Lmt2 function_input; Lmt1 function_input; Value1 function_input; FaultPath1 function_output; FaultPath2 function_output; offset function_input; RelClosing function_output; RelClose function_output; RelOpening function_output; RelClosing function_output; RelClose function_output; RelOpening function_output; I input Bus: I_Current; FaultDet output double =0; FaultElec output Bus: I_Current; CurLmt input Bus: I_Current; Volt input Bus: CellVoltage; Rclosing local double; Ropening local double; FaultTh output Bus: MaxMinLimit; Tp input Bus: MaxMinLimit; BatSt output double; BatReq local; BatSoC input Bus: MaxMinLimit; BatCmd input; Rpos output double; Rneg output double; FaultVolt output Bus: MaxMinLimit; CountFault local double; ThermFault local double; CountCh local double; CountDch local double; CountMax local double; CountMin local double; FaultDisp output Bus: FaultDisp; ElecFault local double =0; VoltFault local double; FaultReset input double; RelChg output double; RelDchg output double; RelChgClosing local double; RelChgOpening local double; RelDchgClosing local double; RelDchgOpening local double; RelDchgClose local double; RelChgClose local double; Rclose local double; MaxVoltLmt parameter double; MinVoltLmt parameter double; MaxThLmt parameter double; MinThLmt parameter double; CurrOffset parameter double; VoltOffset parameter double

== stateflow chart BatteryManagementSystem/Battery Protection Logic/State Flow Logic/Fault Protection/Protection.CurrFault ==
  state FaultDetected
    en,du:
    FaultDet=1;
    ElecFlag=1;
    ElecFault = ...
    duration(ElecFlag==1 ...
    ,msec);
  state NoFault
    en:
    ElecFault=0;
    ElecFlag=0;
  state DebouncePath1
  state FaultCounter
  state DebouncePath2
  (default) -> NoFault : {Count1=0;
      | Count2=0;
      | CountFault=0;
      | FaultPath1=0;
      | FaultPath2=0;
      | FaultDet=0;}
  NoFault -> DebouncePath1 [order 1] : [Value1<Lmt1-offset && Rclose==1]
  DebouncePath1 -> FaultDetected : after(1,sec)
      | {FaultPath1=1;
      | Count1=Count1+1;}
  NoFault -> DebouncePath1 [order 3] : [duration(Value1<Lmt1)>1 ...
      | && Rclose==1]
  FaultCounter -> NoFault [order 1] : [Count1==5 || Count2==5]
      | {CountFault=1;}
  FaultDetected -> FaultCounter : [Rclose==0 ...
      |  && ThermFault==0 ...
      | && ElecFault>=1000]
  FaultCounter -> NoFault [order 2] : {FaultPath1=0;
      | FaultPath2=0;FaultDet=0;}
  NoFault -> DebouncePath2 [order 4] : [duration(Value2>Lmt2)>1 ...
      | && Rclose==1]
  DebouncePath2 -> FaultDetected : after(1,sec)
      | {FaultPath2=1;
      | Count2=Count2+1;}
  NoFault -> DebouncePath2 [order 2] : [Value2>Lmt2+offset && Rclose==1]
  data: FaultDet output double =0; Count1 output double; Count2 output double; ElecFlag output double =0; ElecFault output double =0; CountFault output double; Rclose output double; ThermFault output double; Value2 input; Lmt2 input; Lmt1 input; Value1 input; FaultPath1 output; FaultPath2 output; offset input double

== stateflow chart BatteryManagementSystem/Battery Protection Logic/State Flow Logic/Fault Protection/Protection.VoltageFault ==
  state FaultDetected
    en,du:
    FaultDet=1;
    ElecFlag=1;
    ElecFault = ...
    duration(ElecFlag==1 ...
    ,msec);
  state NoFault
    en:
    ElecFault=0;
    ElecFlag=0;
  state DebouncePath1
  state FaultCounter
  state DebouncePath2
  (default) -> NoFault : {Count1=0;
      | Count2=0;
      | CountFault=0;
      | FaultPath1=0;
      | FaultPath2=0;
      | FaultDet=0;}
  NoFault -> DebouncePath1 [order 1] : [Value1<Lmt1-offset && Rclose==1]
  DebouncePath1 -> FaultDetected : after(1,sec)
      | {FaultPath1=1;
      | Count1=Count1+1;}
  NoFault -> DebouncePath1 [order 3] : [duration(Value1<Lmt1)>1 ...
      | && Rclose==1]
  FaultCounter -> NoFault [order 1] : [Count1==5 || Count2==5]
      | {CountFault=1;}
  FaultDetected -> FaultCounter : [Rclose==0 ...
      |  && ThermFault==0 ...
      | && ElecFault>=1000]
  FaultCounter -> NoFault [order 2] : {FaultPath1=0;
      | FaultPath2=0;FaultDet=0;}
  NoFault -> DebouncePath2 [order 4] : [duration(Value2>Lmt2)>1 ...
      | && Rclose==1]
  DebouncePath2 -> FaultDetected : after(1,sec)
      | {FaultPath2=1;
      | Count2=Count2+1;}
  NoFault -> DebouncePath2 [order 2] : [Value2>Lmt2+offset && Rclose==1]
  data: FaultDet output double =0; Count1 output double; Count2 output double; ElecFlag output double =0; ElecFault output double =0; CountFault output double; Rclose output double; ThermFault output double; Value2 input; Lmt2 input; Lmt1 input; Value1 input; FaultPath1 output; FaultPath2 output; offset input double

== stateflow chart BatteryManagementSystem/Battery Protection Logic/State Flow Logic/Fault Protection/Relay_Charge ==
  state RelayOpen
    state RelayOpen
      Relay=0;
    state Opened
      RelClose=0;
      RelOpening=0;
    (default) -> RelayOpen.RelayOpen
    RelayOpen.RelayOpen -> Opened : after(100,msec)
  state RelayClose
    state PosRelayClose
      Relay=1;
    state Closed
      RelClose=1;
      RelClosing=0;
    (default) -> PosRelayClose
    PosRelayClose -> Closed : after(100,msec)
  (default) -> RelayOpen : {RelClose=0;Relay=0;}
  Opened -> RelayClose : [RelClosing==1]
  Closed -> RelayOpen : [RelOpening==1]
  data: RelClosing output; RelClose output; Relay output; RelOpening output

== stateflow chart BatteryManagementSystem/Battery Protection Logic/State Flow Logic/Fault Protection/Relay_Discharge ==
  state RelayOpen
    state RelayOpen
      Relay=0;
    state Opened
      RelClose=0;
      RelOpening=0;
    (default) -> RelayOpen.RelayOpen
    RelayOpen.RelayOpen -> Opened : after(100,msec)
  state RelayClose
    state PosRelayClose
      Relay=1;
    state Closed
      RelClose=1;
      RelClosing=0;
    (default) -> PosRelayClose
    PosRelayClose -> Closed : after(100,msec)
  (default) -> RelayOpen : {RelClose=0;Relay=0;}
  Opened -> RelayClose : [RelClosing==1]
  Closed -> RelayOpen : [RelOpening==1]
  data: RelClosing output; RelClose output; Relay output; RelOpening output
